simulink model "Calculator"  (R2021b)
settings: Solver=FixedStepDiscrete  StartTime=0.0  StopTime=10.0  RelTol=1e-3  EnableMultiTasking=on
libraries: simulink x2
settings Model: Creator=midol  LastModifiedBy=midol
settings DataIOCC: ReturnWorkspaceOutputs=off
settings OptimizationCC: DefaultParameterBehavior=Inlined  InlineInvariantSignals=on  EnableMemcpy=off  LifeSpan=1  EfficientTunableParamExpr=on
settings DebuggingCC: UnderspecifiedInitializationDetection=Classic  MergeDetectMultiDrivingBlocksExec=none  SFMachineParentedDataDiag=warning  ArithmeticOperatorsInVariantConditions=warning
settings ModelReferenceCC: PropagateSignalLabelsOutOfModel=off
settings SFSimCC: MATLABDynamicMemAlloc=off  CustomCodeUndefinedFunction=UseInterfaceOnly
settings RTWCC: Description=Embedded Coder  SystemTargetFile=ert.tlc  GenCodeOnly=on  TemplateMakefile=ert_default_tmf  GenerateReport=on  IncludeHyperlinkInReport=on  LaunchReport=on  GenerateTraceInfo=on  GenerateTraceReport=on  GenerateTraceReportSl=on  GenerateTraceReportSf=on  GenerateTraceReportEml=on
settings CodeAppCC: ForceParamTrailComments=on  IgnoreCustomStorageClasses=off  OperatorAnnotations=on  SimulinkDataObjDesc=on  SFDataObjDesc=on  MATLABFcnDesc=on  InsertBlockDesc=on  StateflowObjectComments=on  MATLABSourceComments=on
settings ERTTargetCC: MultiwordLength=2048  GenerateSampleERTMain=on  InlinedParameterPlacement=NonHierarchical  ERTCustomFileTemplate=example_file_process.tlc

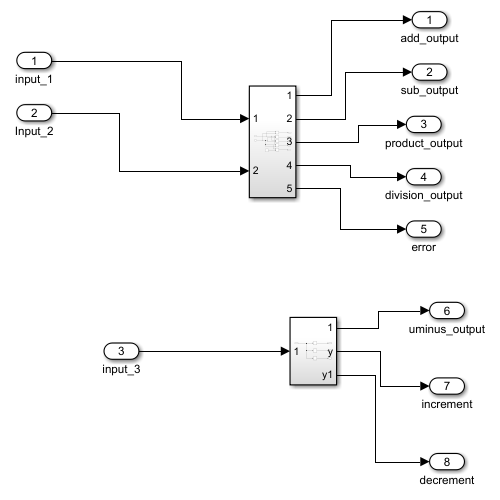
[thumbnail: Simulink's stored preview of the top-level diagram]
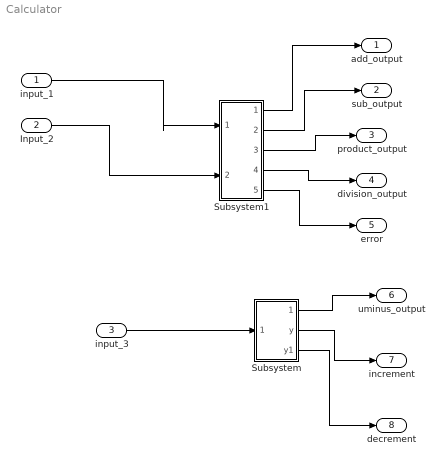
== system Calculator ==
  input_1 : Inport
  Input_2 : Inport  Port=2
  input_3 : Inport  Port=3
  Subsystem : Subsystem
  Subsystem1 : Subsystem
  add_output : Outport
  sub_output : Outport  Port=2
  product_output : Outport  Port=3
  division_output : Outport  Port=4
  error : Outport  Port=5
  uminus_output : Outport  Port=6
  increment : Outport  Port=7
  decrement : Outport  Port=8
  wires:
  input_3/1 -> Subsystem/1(In1)
  Subsystem/1(Out1) -> uminus_output/1
  Subsystem/2(y) -> increment/1
  Subsystem/3(y1) -> decrement/1
  input_1/1 -> Subsystem1/1(In1)
  Input_2/1 -> Subsystem1/2(In2)
  Subsystem1/1(Out1) -> add_output/1
  Subsystem1/2(Out2) -> sub_output/1
  Subsystem1/3(Out3) -> product_output/1
  Subsystem1/4(Out4) -> division_output/1
  Subsystem1/5(Out5) -> error/1

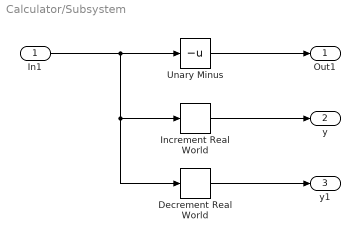
== system Calculator/Subsystem ==
  In1 : Inport
  Decrement Real World : simulink/Additional Math & Discrete/Additional Math: Increment - Decrement/Decrement Real World
      settings: SourceProductBaseCode=SL
  Increment Real World : simulink/Additional Math & Discrete/Additional Math: Increment - Decrement/Increment Real World
      settings: SourceProductBaseCode=SL
  Unary Minus : UnaryMinus
  Out1 : Outport
  y : Outport  Port=2
  y1 : Outport  Port=3
  wires:
  In1/1 -> Decrement Real World/1, Increment Real World/1, Unary Minus/1
  Increment Real World/1 -> y/1
  Decrement Real World/1 -> y1/1
  Unary Minus/1 -> Out1/1

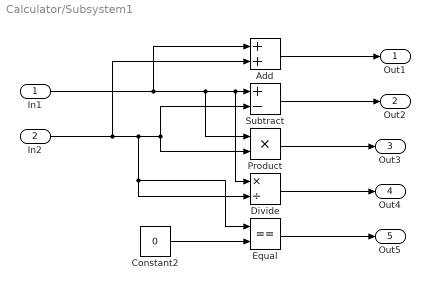
== system Calculator/Subsystem1 ==
  In1 : Inport
  In2 : Inport  Port=2
  Add : Sum
  Constant2 : Constant  Value=0
  Divide : Product  Inputs=*/
  Equal : RelationalOperator  Operator===  OutDataTypeStr=boolean  RndMeth=Simplest
  Product : Product
  Subtract : Sum  Inputs=+-
  Out1 : Outport
  Out2 : Outport  Port=2
  Out3 : Outport  Port=3
  Out4 : Outport  Port=4
  Out5 : Outport  Port=5
  wires:
  Product/1 -> Out3/1
  Equal/1 -> Out5/1
  In2/1 -> Equal/1, Divide/2, Subtract/2, Product/2, Add/2
  Add/1 -> Out1/1
  In1/1 -> Divide/1, Subtract/1, Product/1, Add/1
  Constant2/1 -> Equal/2
  Divide/1 -> Out4/1
  Subtract/1 -> Out2/1
